simulink model "tst_bus_simple_hierarchy"  (Simulink 8.0)
settings: Solver=ode45  StartTime=0.0  StopTime=10.0  RelTol=1e-3
settings Model: Creator=Marci  LastModifiedBy=Marci

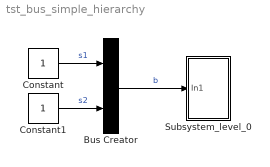
== system tst_bus_simple_hierarchy ==
  Bus Creator : BusCreator  Inputs=2
  Constant : Constant
  Constant1 : Constant
  Subsystem_level_0 : Subsystem
  wires:
  Constant1/1 -> Bus Creator/2  "s2"
  Constant/1 -> Bus Creator/1  "s1"
  Bus Creator/1 -> Subsystem_level_0/1(In1)  "b"

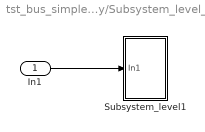
== system tst_bus_simple_hierarchy/Subsystem_level_0 ==
  In1 : Inport
  Subsystem_level1 : Subsystem
  wires:
  In1/1 -> Subsystem_level1/1(In1)

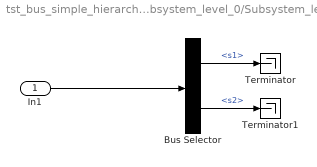
== system tst_bus_simple_hierarchy/Subsystem_level_0/Subsystem_level1 ==
  In1 : Inport
  Bus Selector : BusSelector  OutputSignals=s1,s2
  Terminator : Terminator
  Terminator1 : Terminator
  wires:
  Bus Selector/2 -> Terminator1/1  "<s2>"
  In1/1 -> Bus Selector/1
  Bus Selector/1 -> Terminator/1  "<s1>"
